simulink model "Task1"  (R2020a)
settings: Solver=VariableStepAuto  StartTime=0.0  StopTime=10  MaxStep=1e-3  RelTol=1e-3
settings Model: Creator=dvdia  LastModifiedBy=dvdia

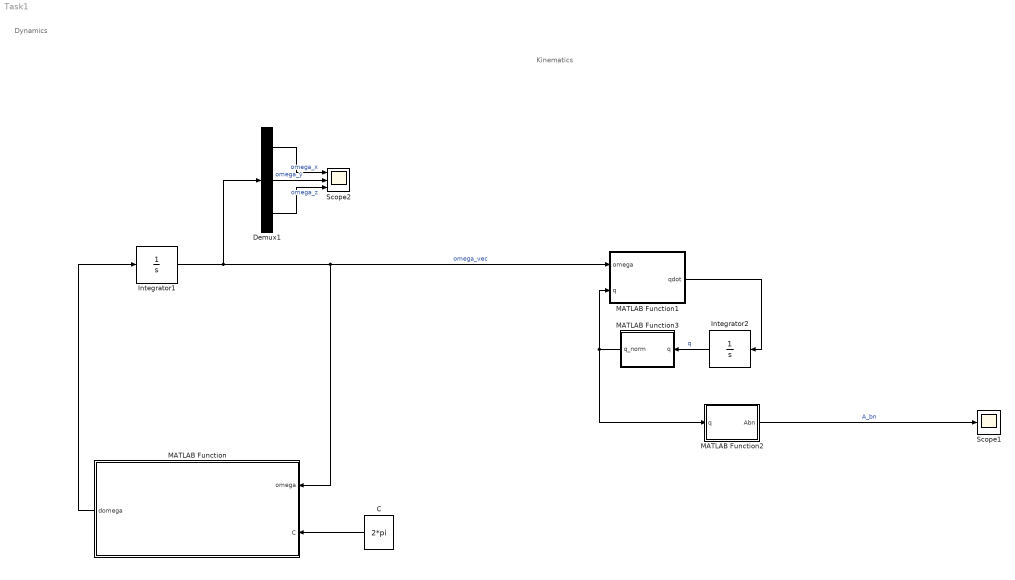
== system Task1 ==
  note: Dynamics
  note: Kinematics
  C : Constant  Value=2*pi
  Demux1 : Demux  Outputs=3
  Integrator1 : Integrator  InitialCondition="[ 2*pi  1.e-2 1e-2]"
  Integrator2 : Integrator  InitialCondition=[ 0 0 0 1]
  MATLAB Function : MATLAB Function  TreatAsAtomicUnit=on
  MATLAB Function1 : MATLAB Function  TreatAsAtomicUnit=on
  MATLAB Function2 : MATLAB Function  TreatAsAtomicUnit=on
  MATLAB Function3 : MATLAB Function  TreatAsAtomicUnit=on
  Scope1 : Scope
  Scope2 : Scope  NumInputPorts=3
  wires:
  Demux1/3 -> Scope2/3  "omega_z"
  Integrator1/1 -> Demux1/1, MATLAB Function1/1(omega), MATLAB Function/1(omega)  "omega_vec"
  Demux1/1 -> Scope2/1  "omega_x"
  C/1 -> MATLAB Function/2(C)
  Demux1/2 -> Scope2/2  "omega_y"
  MATLAB Function/1(domega) -> Integrator1/1
  MATLAB Function1/1(qdot) -> Integrator2/1
  MATLAB Function2/1(Abn) -> Scope1/1  "A_bn"
  Integrator2/1 -> MATLAB Function3/1(q)  "q"
  MATLAB Function3/1(q_norm) -> MATLAB Function2/1(q), MATLAB Function1/2(q)

== matlab function Task1/MATLAB Function ==
  data: omega input; domega output; C input
function domega = fcn(omega,C)

% Inertia moments

I_x = 0.07;         %  [kg*m^2]
I_y = 0.0504;       %  [kg*m^2]
I_z = 0.0109;       %  [kg*m^2]


% Initial conditions

%C = 2*pi;
% C = 0.1;
% C = 1;
% C = 1.5;
% C = 2;
omega0_vec = [C 1.e-2 1e-2];

% Set omegas
omega_x = omega(1);
omega_y = omega(2);
omega_z = omega(3);


% Compute d_omegas
domega_x = (I_y-I_z)*omega_y*omega_z/I_x;
domega_y = (I_z-I_x)*omega_x*omega_z;
domega_z = (I_x - I_y)*omega_y*omega_x / I_z;
domega = [ domega_x domega_y domega_z ];
end

== matlab function Task1/MATLAB Function2 ==
  data: q input; Abn output
function Abn = fcn(q)

Abn = [q(1)^2-q(2)^2-q(3)^2+q(4)^2  2*(q(1)*q(2)+q(3)*q(4))         2*(q(1)*q(3)-q(2)*q(4))
        2*(q(1)*q(2)-q(3)*q(4))     -q(1)^2+q(2)^2-q(3)^2+q(4)^2    2*(q(2)*q(3)+q(1)*q(4))
        2*(q(1)*q(3)+q(2)*q(4))     2*(q(2)*q(3)-q(1)*q(4))         -q(1)^2-q(2)^2+q(3)^2+q(4)^2];
    
end

== matlab function Task1/MATLAB Function3 ==
  data: q input; q_norm output
function q_norm = normalize(q)

q_norm = q./norm(q);

== matlab function Task1/MATLAB Function1 ==
  data: omega input; qdot output; q input
function qdot = kyn_quat(omega,q)

% Kinematics using quaternions

W = [0 omega(3) -omega(2) omega(1)
    -omega(3) 0 omega(1) omega(2)
    omega(2) -omega(1) 0 omega(3)
    - omega(1) -omega(2) -omega(3) 0];

qdot = 1/2 * W *q;
end
